simulink model "Maneuver_wrapper_model"  (R2020a)
settings: Solver=VariableStepAuto  StartTime=0.0  StopTime=10.0  RelTol=1e-3
settings Model: Creator=Matthew  LastModifiedBy=Matthew

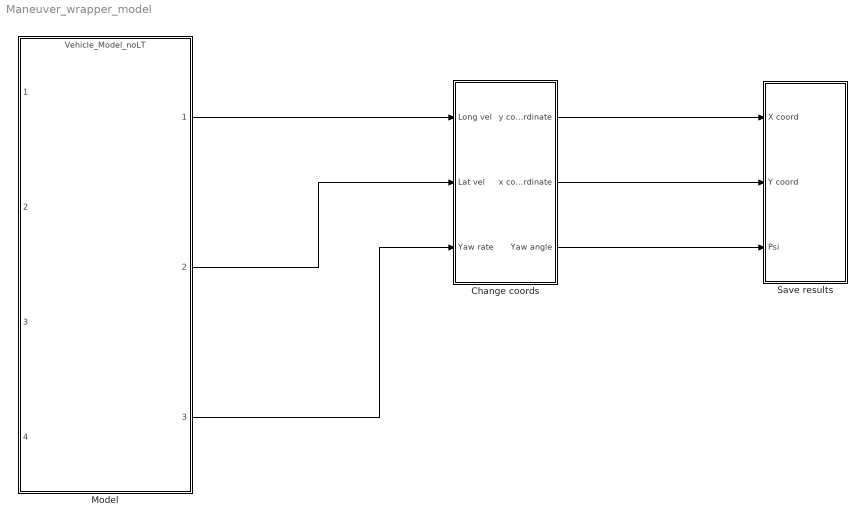
== system Maneuver_wrapper_model ==
  Change coords : Subsystem
  Model : ModelReference  ModelNameDialog=Vehicle_Model_noLT.slx  SimulationMode=Normal  ModelReferenceVersion=1.15
  Save results : Subsystem
  wires:
  Model/1 -> Change coords/1(Long vel)
  Model/2 -> Change coords/2(Lat vel)
  Model/3 -> Change coords/3(Yaw rate)
  Change coords/1(y coordinate) -> Save results/1(X coord)
  Change coords/2(x coordinate) -> Save results/2(Y coord)
  Change coords/3(Yaw angle) -> Save results/3(Psi)

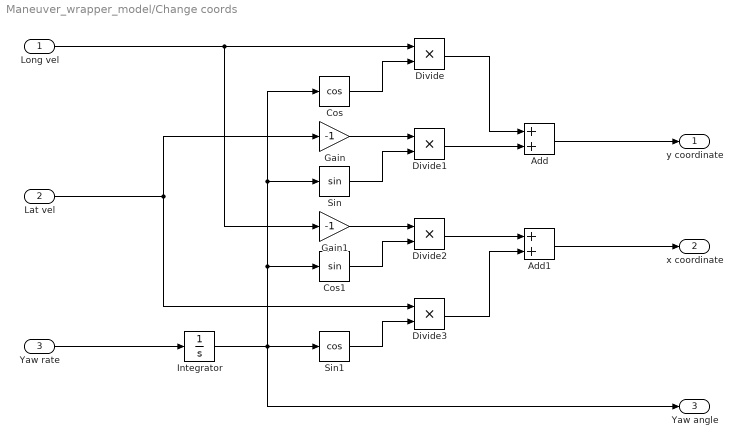
== system Maneuver_wrapper_model/Change coords ==
  Long vel : Inport
  Lat vel : Inport  Port=2
  Yaw rate : Inport  Port=3
  Add : Sum
  Add1 : Sum
  Cos : Trigonometry  Operator=cos
  Cos1 : Trigonometry
  Divide{,1..3} (4 alike) : Product  Inputs=**
  Gain : Gain  Gain=-1
  Gain1 : Gain  Gain=-1
  Integrator : Integrator
  Sin : Trigonometry
  Sin1 : Trigonometry  Operator=cos
  y coordinate : Outport
  x coordinate : Outport  Port=2
  Yaw angle : Outport  Port=3
  wires:
  Gain/1 -> Divide1/1
  Integrator/1 -> Yaw angle/1, Sin/1, Cos/1, Cos1/1, Sin1/1
  Sin/1 -> Divide1/2
  Gain1/1 -> Divide2/1
  Divide3/1 -> Add1/2
  Sin1/1 -> Divide3/2
  Divide1/1 -> Add/2
  Yaw rate/1 -> Integrator/1
  Add1/1 -> x coordinate/1
  Long vel/1 -> Gain1/1, Divide/1
  Divide2/1 -> Add1/1
  Divide/1 -> Add/1
  Lat vel/1 -> Gain/1, Divide3/1
  Cos/1 -> Divide/2
  Cos1/1 -> Divide2/2
  Add/1 -> y coordinate/1

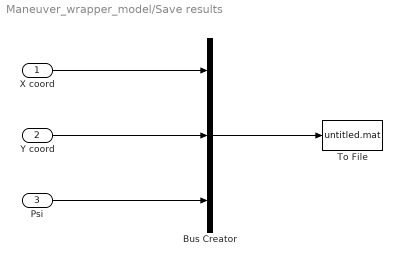
== system Maneuver_wrapper_model/Save results ==
  X coord : Inport
  Y coord : Inport  Port=2
  Psi : Inport  Port=3
  Bus Creator : BusCreator  Inputs=3
  To File : ToFile  SaveFormat=Timeseries
  wires:
  X coord/1 -> Bus Creator/1
  Y coord/1 -> Bus Creator/2
  Psi/1 -> Bus Creator/3
  Bus Creator/1 -> To File/1
